simulink model "psbtransfo3wdn"  (Simulink 6.0)
settings: Solver=ode15s  StartTime=0.0  StopTime=10.0  RelTol=1e-3
InitFcn:
  | powericon('psbinitsys',bdroot);
undefined symbols (not defined in the file or in its folder): D1, Delta
libraries: powerlib2 x28
settings Model: Creator=patrice  LastModifiedBy=batserve  ExtModeTrigMode=oneshot  ExtModeArmWhenConnect=off  ExtModeAutoUpdateStatusClock=off
settings DataIOCC: LimitDataPoints=off  SignalLoggingName=sigsOut
settings OptimizationCC: BooleanDataType=off
settings DebuggingCC: SolverPrmCheckMsg=none
settings HardwareCC: TargetUnknown=on

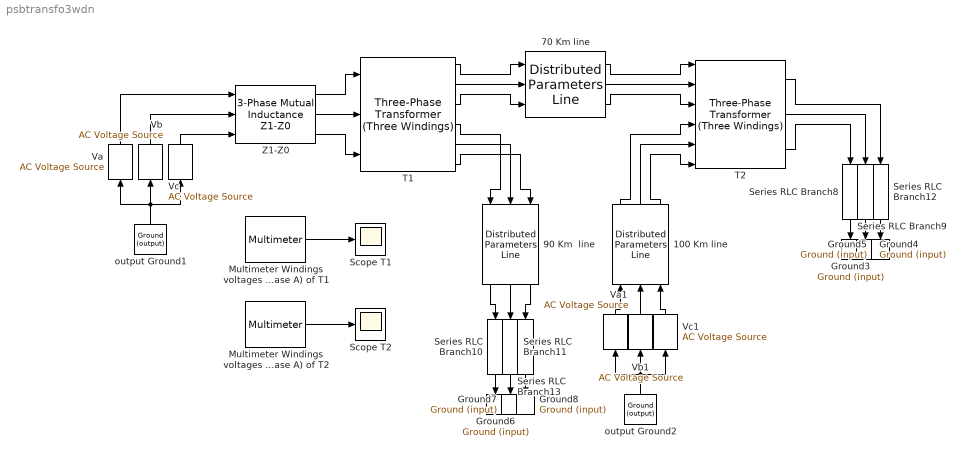
== system psbtransfo3wdn ==
  100 Km line : powerlib2/Elements/Distributed Parameters Line  Tag=PoWeRsYsTeMbLoCk  Orientation=up  n=3  f=60  r=[0.045 0.383]  l="[0.0009536  .0034]"  c="[12.02e-9   7.47e-9]"  lgt=100  x1=[0 0.7635 6.552e+04 -3.356e+05;0.0004716 0.2984 1.238e+05 -3.187e+05;0.0009433 -0.1761 1.782e+05 -2.918e+05;0.001415 -0.645 2.27e+05 -2.556e+05;0.001887 -1.094 2.687e+05 -2.114e+05;0.002358 -1.508 3.018e+05 -1.606e+05]  x2=[0 1.583 2.165e+04 -3.402e+05;0.0004716 0.789 8.149e+04 -3.31e+05;0.0009433 -0.02989 1.388e+05 -3.114e+05;0.001415 -0.8479 1.916e+05 -2.82e+05;0.001887 -1.639 2.385e+05 -2.436e+05;0.002358 -2.379 2.778e+05 -1.976e+05]  x3=[0 0.02395 -235.2 649.9;0.0004716 0.02363 -346.5 598;0.0009433 0.02255 -446.8 527.3;0.001415 0.02077 -533 440;0.001887 0.01833 -602.4 338.8;0.002358 0.01531 -652.8 226.9]  x4=[0 -0.01995 443.3 -3029;0.0004716 -0.02141 972 -2902;0.0009433 -0.02221 1470 -2685;0.001415 -0.0223 1922 -2382;0.001887 -0.02169 2313 -2005;0.002358 -0.02039 2631 -1564]  x5=0.002358  mesure=None  PSBOutputType=111111111111111111111111111111
  70 Km line : powerlib2/Elements/Distributed Parameters Line  Tag=PoWeRsYsTeMbLoCk  n=3  f=60  r=[0.045 0.383]  l="[0.0009536  .0034]"  c="[12.02e-9   7.47e-9]"  lgt=70  x1=[0 0.7635 6.552e+04 -3.356e+05;0.0004716 0.2984 1.238e+05 -3.187e+05;0.0009433 -0.1761 1.782e+05 -2.918e+05;0.001415 -0.645 2.27e+05 -2.556e+05;0.001887 -1.094 2.687e+05 -2.114e+05;0.002358 -1.508 3.018e+05 -1.606e+05]  x2=[0 1.583 2.165e+04 -3.402e+05;0.0004716 0.789 8.149e+04 -3.31e+05;0.0009433 -0.02989 1.388e+05 -3.114e+05;0.001415 -0.8479 1.916e+05 -2.82e+05;0.001887 -1.639 2.385e+05 -2.436e+05;0.002358 -2.379 2.778e+05 -1.976e+05]  x3=[0 0.02395 -235.2 649.9;0.0004716 0.02363 -346.5 598;0.0009433 0.02255 -446.8 527.3;0.001415 0.02077 -533 440;0.001887 0.01833 -602.4 338.8;0.002358 0.01531 -652.8 226.9]  x4=[0 -0.01995 443.3 -3029;0.0004716 -0.02141 972 -2902;0.0009433 -0.02221 1470 -2685;0.001415 -0.0223 1922 -2382;0.001887 -0.02169 2313 -2005;0.002358 -0.02039 2631 -1564]  x5=0.002358  mesure=None  PSBOutputType=111111111111111111111111111111
  90 Km  line : powerlib2/Elements/Distributed Parameters Line  Tag=PoWeRsYsTeMbLoCk  Orientation=down  n=3  f=60  r=[0.045 0.383]  l="[0.0009536  .0034]"  c="[12.02e-9   7.47e-9]"  lgt=90  x1=[0 0.7635 6.552e+04 -3.356e+05;0.0004716 0.2984 1.238e+05 -3.187e+05;0.0009433 -0.1761 1.782e+05 -2.918e+05;0.001415 -0.645 2.27e+05 -2.556e+05;0.001887 -1.094 2.687e+05 -2.114e+05;0.002358 -1.508 3.018e+05 -1.606e+05]  x2=[0 1.583 2.165e+04 -3.402e+05;0.0004716 0.789 8.149e+04 -3.31e+05;0.0009433 -0.02989 1.388e+05 -3.114e+05;0.001415 -0.8479 1.916e+05 -2.82e+05;0.001887 -1.639 2.385e+05 -2.436e+05;0.002358 -2.379 2.778e+05 -1.976e+05]  x3=[0 0.02395 -235.2 649.9;0.0004716 0.02363 -346.5 598;0.0009433 0.02255 -446.8 527.3;0.001415 0.02077 -533 440;0.001887 0.01833 -602.4 338.8;0.002358 0.01531 -652.8 226.9]  x4=[0 -0.01995 443.3 -3029;0.0004716 -0.02141 972 -2902;0.0009433 -0.02221 1470 -2685;0.001415 -0.0223 1922 -2382;0.001887 -0.02169 2313 -2005;0.002358 -0.02039 2631 -1564]  x5=0.002358  mesure=None  PSBOutputType=111111111111111111111111111111
  Ground{3..8} (6 alike) : powerlib2/Connectors/Ground (input)  Tag=PoWeRsYsTeMbLoCk  Orientation=down
  Multimeter Windings voltages (phase A) of T1 : powerlib2/Measurements/Multimeter  Tag=PoWeRsYsTeMmEaSuReMeNt  PhasorSimulation=off  OutputType=Magnitude  sel=[1 4 7]  L=18  Gain=[1 1 1]  yselected=[511,8.4485067260742188e+004;512,8.4485067260742188e+004;313,8.4485067260742188e+004]  PSBOutputType=1  PSBequivalent=0  AxesSetting=[0,0.1,-100,100]  Display=0  SavedBlockNames={}
  Multimeter Windings voltages (phase A) of T2 : powerlib2/Measurements/Multimeter  Tag=PoWeRsYsTeMmEaSuReMeNt  PhasorSimulation=off  OutputType=Magnitude  sel=[10 13 16]  L=18  Gain=[1 1 1]  yselected=[411,8.4486067260742188e+004;412,8.4486067260742188e+004;313,8.4486067260742188e+004]  PSBOutputType=1  PSBequivalent=0  AxesSetting=[0,0.1,-100,100]  Display=0  SavedBlockNames={}
  Scope T1 : Scope
      settings: TimeRange=0.1  YMin=-400000  YMax=400000
  Scope T2 : Scope
      settings: TimeRange=0.1  YMin=-1000000  YMax=1000000
  Series RLC Branch{8..13} (6 alike) : powerlib2/Elements/Series RLC Branch  Tag=PoWeRsYsTeMbLoCk  Orientation=down  a=5.7  b=6.03  c=inf  mesure=None  PSBOutputType=1
  T1 : powerlib2/Elements/Three-Phase Transformer (Three Windings)  Tag=PoWeRsYsTeMbLoCk  confi=ABC as input terminals  nom=[ 250e6 , 60 ]  ydw1=Yg  w1=[ 735e3 , 0.002 , 0.08 ]  ydw2=Yg  w2=[ 315e3 , 0.002 , 0.08 ]  ydw3=Delta (D1)  w3=[ 315e3 , 0.002 , 0.08 ]  ynsat=off  rmag=500  lm=500  sat="[ 0,0  ;  0.005,1.2  ;  1.0,1.4]"  hyst=off  matfile='hysteresis'  sif=off  ifl=[0.8 -0.8 0.7]  initialslopes=[+1 +1 +1]  mesure=Winding voltages  PSBOutputType=1111111
  T2 : powerlib2/Elements/Three-Phase Transformer (Three Windings)  Tag=PoWeRsYsTeMbLoCk  confi=ABC as output terminals  nom=[ 250e6 , 60 ]  ydw1=Y  w1=[ 735e3 , 0.002 , 0.08 ]  ydw2=Y  w2=[ 315e3 , 0.002 , 0.08 ]  ydw3=Delta (D1)  w3=[ 315e3 , 0.002 , 0.08 ]  ynsat=off  rmag=500  lm=500  sat="[ 0,0  ;  0.005,1.2  ;  1.0,1.4]"  hyst=off  matfile='hysteresis'  sif=off  ifl=[0.8 -0.8 0.7]  initialslopes=[+1 +1 +1]  mesure=Winding voltages  PSBOutputType=1111111
  Va : powerlib2/Electrical Sources/AC Voltage Source  Tag=PoWeRsYsTeMbLoCk  Orientation=up  A=315e3  P=-65.4  F=60  stime=0  mesure=None  PSBOutputType=1
  Va1 : powerlib2/Electrical Sources/AC Voltage Source  Tag=PoWeRsYsTeMbLoCk  Orientation=up  A=479690  P=0  F=60  stime=0  mesure=None  PSBOutputType=1
  Vb : powerlib2/Electrical Sources/AC Voltage Source  Tag=PoWeRsYsTeMbLoCk  Orientation=up  A=315e3  P=-65.4-120  F=60  stime=0  mesure=None  PSBOutputType=1
  Vb1 : powerlib2/Electrical Sources/AC Voltage Source  Tag=PoWeRsYsTeMbLoCk  Orientation=up  A=470000  P=-120  F=60  stime=0  mesure=None  PSBOutputType=1
  Vc : powerlib2/Electrical Sources/AC Voltage Source  Tag=PoWeRsYsTeMbLoCk  Orientation=up  A=479690  P=-65.4+120  F=60  stime=0  mesure=None  PSBOutputType=1
  Vc1 : powerlib2/Electrical Sources/AC Voltage Source  Tag=PoWeRsYsTeMbLoCk  Orientation=up  A=470000  P=+120  F=60  stime=0  mesure=None  PSBOutputType=1
  Z1-Z0 : powerlib2/Elements/3-Phase Mutual Inductance Z1-Z0  RL1="[ 2  50e-3]"  RL0="[4  100e-3]"
  output Ground1 : powerlib2/Connectors/Ground (output)  Tag=PoWeRsYsTeMbLoCk  Orientation=up  PSBOutputType=1
  output Ground2 : powerlib2/Connectors/Ground (output)  Tag=PoWeRsYsTeMbLoCk  Orientation=up  PSBOutputType=1
  wires:
  T1/2 -> 70 Km line/2
  T1/3 -> 70 Km line/3
  T1/1 -> 70 Km line/1
  T2/3 -> Series RLC Branch8/1
  T2/2 -> Series RLC Branch9/1
  T2/1 -> Series RLC Branch12/1
  70 Km line/2 -> T2/2
  70 Km line/1 -> T2/1
  70 Km line/3 -> T2/3
  Series RLC Branch8/1 -> Ground3/1
  Series RLC Branch9/1 -> Ground4/1
  Series RLC Branch12/1 -> Ground5/1
  T1/4 -> 90 Km  line/1
  T1/5 -> 90 Km  line/2
  T1/6 -> 90 Km  line/3
  Z1-Z0/1 -> T1/1
  Z1-Z0/2 -> T1/2
  Z1-Z0/3 -> T1/3
  Vc/1 -> Z1-Z0/3
  Vb/1 -> Z1-Z0/2
  Va/1 -> Z1-Z0/1
  output Ground1/1 -> Vc/1, Va/1, Vb/1
  Series RLC Branch10/1 -> Ground6/1
  Series RLC Branch11/1 -> Ground7/1
  Series RLC Branch13/1 -> Ground8/1
  90 Km  line/2 -> Series RLC Branch11/1
  90 Km  line/3 -> Series RLC Branch13/1
  90 Km  line/1 -> Series RLC Branch10/1
  100 Km line/3 -> T2/6
  100 Km line/2 -> T2/5
  100 Km line/1 -> T2/4
  output Ground2/1 -> Vb1/1, Va1/1, Vc1/1
  Vb1/1 -> 100 Km line/2
  Va1/1 -> 100 Km line/1
  Vc1/1 -> 100 Km line/3
  Multimeter Windings voltages (phase A) of T1/1 -> Scope T1/1
  Multimeter Windings voltages (phase A) of T2/1 -> Scope T2/1
